simulink model "ADIP_LocalSim"  (R2019a)
settings: Solver=FixedStepAuto  StartTime=0.0  StopTime=param.Tsim  FixedStep=param.Ts  MaxStep=0.2  RelTol=1e-3
values from neighbouring files (symbols this model uses):
  At = param.A_uu    [runLocalModel.m]
  Fi_t = -lqi(syst_D,Qi,R)    [runLocalModel.m]
  Ft = -dlqr(syst_D.A,syst_D.B,Q,R)    [runLocalModel.m]
undefined symbols (not defined in the file or in its folder): param, sigbuilder_block
settings Model: Creator=yashasvi_sai  LastModifiedBy=ICS
settings SolverCC: ZeroCrossAlgorithm=Adaptive
settings DebuggingCC: IgnoredZcDiagnostic=none

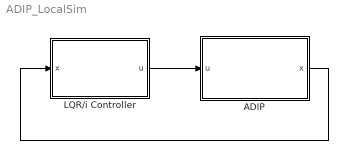
== system ADIP_LocalSim ==
  ADIP : Subsystem
  LQR/i Controller : Subsystem
  wires:
  LQR/i Controller/1(u) -> ADIP/1(u)
  ADIP/1(x) -> LQR/i Controller/1(x)

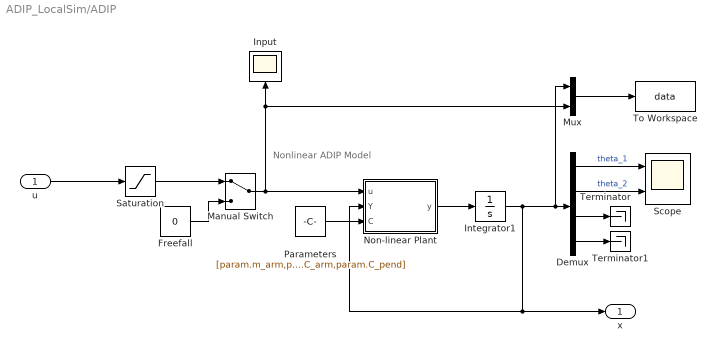
== system ADIP_LocalSim/ADIP ==
  note: Nonlinear ADIP Model
  u : Inport
  Demux : Demux
  Freefall : Constant  Value=0
  Input : Scope
  Integrator1 : Integrator  InitialCondition=param.theta0
  Manual Switch : ManualSwitch
  Mux : Mux  Inputs=2
  "Non-linear Plant " : MATLAB Function  TreatAsAtomicUnit=on
  Parameters : Constant  Value=[param.m_arm,param.m_pend,param.m_hinge,param.l_pivot,param.l_pend,param.g,param.Jarm,param.Jpend,param.Jl,param.Jhinge, param.C_arm,param.C_pend]
  Saturation : Saturate  UpperLimit=2.5  LowerLimit=-2.5
  Scope : Scope  NumInputPorts=2
  Terminator : Terminator
  Terminator1 : Terminator
  To Workspace : ToWorkspace  VariableName=data  SampleTime=-1
  x : Outport
  wires:
  Demux/2 -> Scope/2  "theta_2"
  Demux/4 -> Terminator1/1
  Integrator1/1 -> Mux/1, Demux/1, "Non-linear Plant "/2(Y), x/1
  Mux/1 -> To Workspace/1
  "Non-linear Plant "/1(y) -> Integrator1/1
  Manual Switch/1 -> "Non-linear Plant "/1(u), Mux/2, Input/1
  Demux/1 -> Scope/1  "theta_1"
  Saturation/1 -> Manual Switch/1
  Freefall/1 -> Manual Switch/2
  Demux/3 -> Terminator/1
  Parameters/1 -> "Non-linear Plant "/3(C)
  u/1 -> Saturation/1

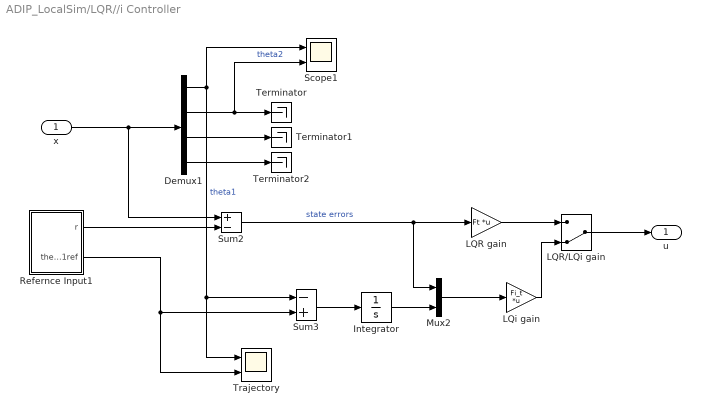
== system ADIP_LocalSim/LQR//i Controller ==
  x : Inport
  Demux1 : Demux
  Integrator : Integrator
  LQR gain : Gain  Gain=Ft  Multiplication=Matrix(K*u)
  LQR/LQi gain : ManualSwitch  CurrentSetting=0
  LQi gain : Gain  Gain=Fi_t  Multiplication=Matrix(K*u)
  Mux2 : Mux  Inputs=2
  Refernce Input1 : Subsystem
  Scope1 : Scope  NumInputPorts=2
  Sum2 : Sum  Inputs=+-
  Sum3 : Sum  Inputs=-+
  Terminator : Terminator
  Terminator1 : Terminator
  Terminator2 : Terminator
  Trajectory : Scope  NumInputPorts=2
  u : Outport
  wires:
  Refernce Input1/2(theta1ref) -> Trajectory/2, Sum3/2
  Mux2/1 -> LQi gain/1
  Demux1/4 -> Terminator2/1
  Demux1/2 -> Terminator/1, Scope1/2  "theta2"
  Demux1/3 -> Terminator1/1
  LQR gain/1 -> LQR/LQi gain/1
  LQi gain/1 -> LQR/LQi gain/2
  LQR/LQi gain/1 -> u/1
  Sum3/1 -> Integrator/1
  Refernce Input1/1(r) -> Sum2/2
  Sum2/1 -> Mux2/1, LQR gain/1  "state errors"
  Integrator/1 -> Mux2/2
  Demux1/1 -> Trajectory/1, Sum3/1, Scope1/1  "theta1"
  x/1 -> Sum2/1, Demux1/1

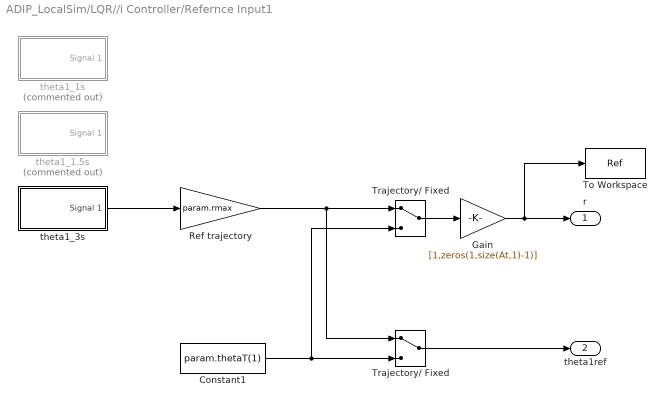
== system ADIP_LocalSim/LQR//i Controller/Refernce Input1 ==
  Constant1 : Constant  Value=param.thetaT(1)
  Gain : Gain  Gain=[1,zeros(1,size(At,1)-1)]
  Ref trajectory : Gain  Gain=param.rmax
  To Workspace : ToWorkspace  VariableName=Ref  SampleTime=-1
  "Trajectory/ Fixed " : ManualSwitch
  Trajectory/ Fixed : ManualSwitch
  theta1_1.5s : Subsystem  Tag=STV Subsys  Commented=on  LoadFcn=sigbuilder_block('load');  StartFcn=sigbuilder_block('start');  StopFcn=sigbuilder_block('stop');  ClipboardFcn=sigbuilder_block('clipboard');  mask(Sigbuilder block){tuvar=[0:10]}
      mask help: Simulink:masks:SigbuilderBlock_MD
      mask init:
      | if ~strcmp(get_param(bdroot(gcbh),'SimulationStatus'),'stopped') tuvar = sigbuilder_block('maskInit'); end
      settings: CopyFcn=sigbuilder_block('copy');  DeleteFcn=sigbuilder_block('delete');  ModelCloseFcn=sigbuilder_block('modelClose');  PreSaveFcn=sigbuilder_block('preSave');  PauseFcn=sigbuilder_block('pause');  ContinueFcn=sigbuilder_block('continue');  NameChangeFcn=sigbuilder_block('namechange');  OpenFcn=sigbuilder_block('open',[5.5 30 1909 958 ]);  CloseFcn=sigbuilder_block('close');
      mask Display: plot(0, 0, 100, 100,[2, 2, 32, 32, 2], [68, 8, 8, 68, 68],[32, 2], [38, 38], [32, 19, 2],[53, 60, 44], [32, 17, 17, 2],[16, 16, 31, 31]);txt = getActiveGroup(gcbh);text(2, 100, txt,'verticalAlignment', 'top');
  theta1_1s : Subsystem  Tag=STV Subsys  Commented=on  LoadFcn=sigbuilder_block('load');  StartFcn=sigbuilder_block('start');  StopFcn=sigbuilder_block('stop');  ClipboardFcn=sigbuilder_block('clipboard');  mask(Sigbuilder block){tuvar=[0:10]}
      mask help: Simulink:masks:SigbuilderBlock_MD
      mask init:
      | if ~strcmp(get_param(bdroot(gcbh),'SimulationStatus'),'stopped') tuvar = sigbuilder_block('maskInit'); end
      settings: CopyFcn=sigbuilder_block('copy');  DeleteFcn=sigbuilder_block('delete');  ModelCloseFcn=sigbuilder_block('modelClose');  PreSaveFcn=sigbuilder_block('preSave');  PauseFcn=sigbuilder_block('pause');  ContinueFcn=sigbuilder_block('continue');  NameChangeFcn=sigbuilder_block('namechange');  OpenFcn=sigbuilder_block('open',[5.5 30 1909 958 ]);  CloseFcn=sigbuilder_block('close');
      mask Display: plot(0, 0, 100, 100,[2, 2, 32, 32, 2], [68, 8, 8, 68, 68],[32, 2], [38, 38], [32, 19, 2],[53, 60, 44], [32, 17, 17, 2],[16, 16, 31, 31]);txt = getActiveGroup(gcbh);text(2, 100, txt,'verticalAlignment', 'top');
  theta1_3s : Subsystem  Tag=STV Subsys  LoadFcn=sigbuilder_block('load');  StartFcn=sigbuilder_block('start');  StopFcn=sigbuilder_block('stop');  ClipboardFcn=sigbuilder_block('clipboard');  mask(Sigbuilder block){tuvar=[0:10]}
      mask help: Simulink:masks:SigbuilderBlock_MD
      mask init:
      | if ~strcmp(get_param(bdroot(gcbh),'SimulationStatus'),'stopped') tuvar = sigbuilder_block('maskInit'); end
      settings: CopyFcn=sigbuilder_block('copy');  DeleteFcn=sigbuilder_block('delete');  ModelCloseFcn=sigbuilder_block('modelClose');  PreSaveFcn=sigbuilder_block('preSave');  PauseFcn=sigbuilder_block('pause');  ContinueFcn=sigbuilder_block('continue');  NameChangeFcn=sigbuilder_block('namechange');  OpenFcn=sigbuilder_block('open',[5.5 30 1909 958 ]);  CloseFcn=sigbuilder_block('close');
      mask Display: plot(0, 0, 100, 100,[2, 2, 32, 32, 2], [68, 8, 8, 68, 68],[32, 2], [38, 38], [32, 19, 2],[53, 60, 44], [32, 17, 17, 2],[16, 16, 31, 31]);txt = getActiveGroup(gcbh);text(2, 100, txt,'verticalAlignment', 'top');
  r : Outport
  theta1ref : Outport  Port=2
  wires:
  Gain/1 -> To Workspace/1, r/1
  Constant1/1 -> Trajectory/ Fixed/2, "Trajectory/ Fixed "/2
  Trajectory/ Fixed/1 -> theta1ref/1
  "Trajectory/ Fixed "/1 -> Gain/1
  Ref trajectory/1 -> Trajectory/ Fixed/1, "Trajectory/ Fixed "/1
  theta1_3s/1(Signal 1) -> Ref trajectory/1

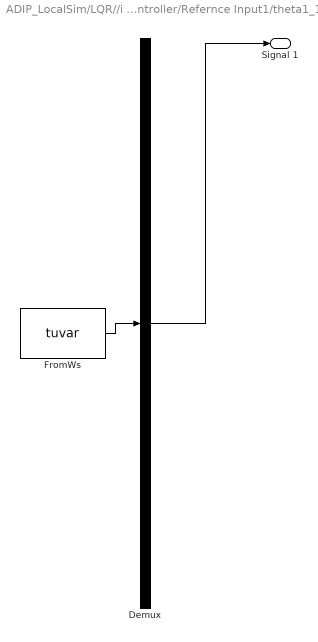
== system ADIP_LocalSim/LQR//i Controller/Refernce Input1/theta1_1.5s ==
  Demux : Demux  Tag=STV Demux  Outputs=1
  FromWs : FromWorkspace  Tag=STV FromWs  VariableName=tuvar  SampleTime=0
      SigBuilderData=|
      | common.afterFinalStr = 'Extrapolate'
      | common.sampleTime = 0
      | dataSet.timeRange = [0 50]
      | dataSet.name = 'Group 1'
      | sbobj.Groups.Name = 'Group 1'
      | sbobj.Groups.Signals.Name = 'Signal 1'
      | sbobj.Groups.Signals.XData = [0 2 3.5 6.5 9.5 12.5 14 50]
      | sbobj.Groups.Signals.YData = [0 0 1 1 -1 -1 0 0]
      | sbobj.Groups.TimeRange = [0 50]
  Signal 1 : Outport  Tag=STV Outport
  wires:
  Demux/1 -> Signal 1/1
  FromWs/1 -> Demux/1

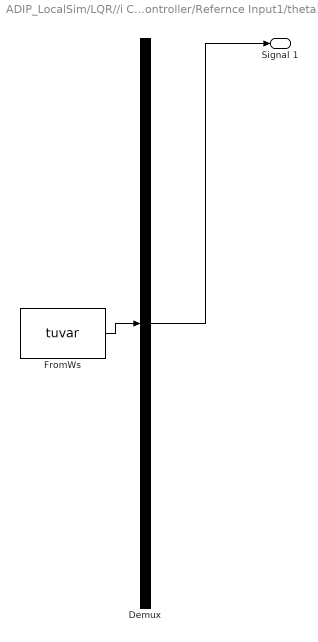
== system ADIP_LocalSim/LQR//i Controller/Refernce Input1/theta1_1s ==
  Demux : Demux  Tag=STV Demux  Outputs=1
  FromWs : FromWorkspace  Tag=STV FromWs  VariableName=tuvar  SampleTime=0
      SigBuilderData=|
      | common.afterFinalStr = 'Extrapolate'
      | common.sampleTime = 0
      | dataSet.timeRange = [0 50]
      | dataSet.name = 'Group 1'
      | sbobj.Groups.Name = 'Group 1'
      | sbobj.Groups.Signals.Name = 'Signal 1'
      | sbobj.Groups.Signals.XData = [0 2 3 6.5 8.5 12.5 13.5 50]
      | sbobj.Groups.Signals.YData = [0 0 1 1 -1 -1 0 0]
      | sbobj.Groups.TimeRange = [0 50]
  Signal 1 : Outport  Tag=STV Outport
  wires:
  Demux/1 -> Signal 1/1
  FromWs/1 -> Demux/1

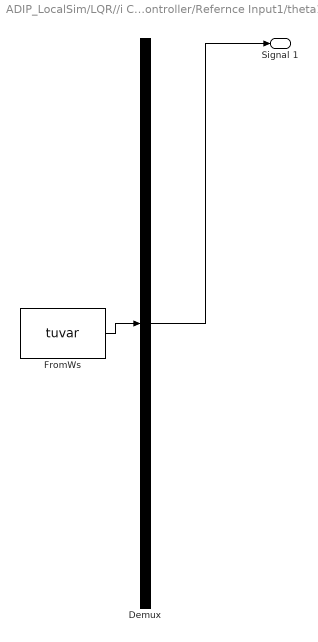
== system ADIP_LocalSim/LQR//i Controller/Refernce Input1/theta1_3s ==
  Demux : Demux  Tag=STV Demux  Outputs=1
  FromWs : FromWorkspace  Tag=STV FromWs  VariableName=tuvar  SampleTime=0
      SigBuilderData=|
      | common.afterFinalStr = 'Extrapolate'
      | common.sampleTime = 0
      | dataSet.timeRange = [0 50]
      | dataSet.name = 'Group 1'
      | sbobj.Groups.Name = 'Group 1'
      | sbobj.Groups.Signals.Name = 'Signal 1'
      | sbobj.Groups.Signals.XData = [0 2 5 6.5 10.5 12 15 50]
      | sbobj.Groups.Signals.YData = [0 0 1 1 -1 -1 0 0]
      | sbobj.Groups.TimeRange = [0 50]
  Signal 1 : Outport  Tag=STV Outport
  wires:
  Demux/1 -> Signal 1/1
  FromWs/1 -> Demux/1

== matlab function ADIP_LocalSim/ADIP/Non-linear Plant  ==
  data: u input; Y input; y output; C input
function y = fcn(u,Y,C)
m1=C(1); % Mass of arm
m2=C(2); % Mass of pendulum
mh = C(3); % Mass of Hinge
l1  = C(4); % Length of arm
l2 = C(5); % Length of pendulum
g_ = C(6);
J_arm = C(7);
J_pend = C(8);
J_motor = C(9);
J_sensor = C(10);
fv1 = C(11);
fv2 = C(12);

y1 = Y(1);  % actual theta1          
y2 = Y(2);  % actual theta2
y3 = Y(3);  % actual theta1d
y4 = Y(4);  % actual theta2d

dy1 = y3;
dy2 = y4;
dy3 =-(2*(8*J_pend*fv1*y3 - 2*l2^2*m2*u - 8*J_pend*u + 2*fv1*l2^2*m2*y3 + l1^2*l2^2*m2^2*y3^2*sin(2*y1 - 2*y2) + l1*l2^3*m2^2*y4^2*sin(y1 - y2) + g_*l1*l2^2*m2^2*sin(y1) + 4*J_pend*g_*l1*m1*sin(y1) + 8*J_pend*g_*l1*m2*sin(y1) + 8*J_pend*g_*l1*mh*sin(y1) + g_*l1*l2^2*m2^2*sin(y1 - 2*y2) - 4*fv2*l1*l2*m2*y4*cos(y1 - y2) + g_*l1*l2^2*m1*m2*sin(y1) + 2*g_*l1*l2^2*m2*mh*sin(y1) + 4*J_pend*l1*l2*m2*y4^2*sin(y1 - y2)))/(16*J_arm*J_pend + 16*J_motor*J_pend + 16*J_pend*J_sensor + 4*l1^2*l2^2*m2^2 + 4*J_arm*l2^2*m2 + 4*J_motor*l2^2*m2 + 4*J_pend*l1^2*m1 + 16*J_pend*l1^2*m2 + 4*J_sensor*l2^2*m2 - 4*l1^2*l2^2*m2^2*cos(y1 - y2)^2 + l1^2*l2^2*m1*m2);
dy4 =(2*(l1^2*l2^2*m2^2*y4^2*sin(2*y1 - 2*y2) - 8*J_motor*fv2*y4 - 8*J_sensor*fv2*y4 - 2*fv2*l1^2*m1*y4 - 8*fv2*l1^2*m2*y4 - 8*J_arm*fv2*y4 - 4*l1*l2*m2*u*cos(y1 - y2) + 2*g_*l1^2*l2*m2^2*sin(2*y1 - y2) + 4*l1^3*l2*m2^2*y3^2*sin(y1 - y2) - 2*g_*l1^2*l2*m2^2*sin(y2) - 4*J_arm*g_*l2*m2*sin(y2) - 4*J_motor*g_*l2*m2*sin(y2) - 4*J_sensor*g_*l2*m2*sin(y2) + g_*l1^2*l2*m1*m2*sin(2*y1 - y2) + 2*g_*l1^2*l2*m2*mh*sin(2*y1 - y2) + l1^3*l2*m1*m2*y3^2*sin(y1 - y2) + 4*fv1*l1*l2*m2*y3*cos(y1 - y2) + 2*g_*l1^2*l2*m2*mh*sin(y2) + 4*J_arm*l1*l2*m2*y3^2*sin(y1 - y2) + 4*J_motor*l1*l2*m2*y3^2*sin(y1 - y2) + 4*J_sensor*l1*l2*m2*y3^2*sin(y1 - y2)))/(16*J_arm*J_pend + 16*J_motor*J_pend + 16*J_pend*J_sensor + 2*l1^2*l2^2*m2^2 + 4*J_arm*l2^2*m2 + 4*J_motor*l2^2*m2 + 4*J_pend*l1^2*m1 + 16*J_pend*l1^2*m2 + 4*J_sensor*l2^2*m2 - 2*l1^2*l2^2*m2^2*cos(2*y1 - 2*y2) + l1^2*l2^2*m1*m2);
y = [dy1 dy2 dy3 dy4]';
